simulink model "F16ASYM_Controlled"  (R2015a)
settings: Solver=ode3  SolverMode=SingleTasking  StartTime=0.0  StopTime=inf  FixedStep=T_sim  RelTol=1e-3
InitFcn:
  | load('NN_c_weights_Last_stable.mat')
StopFcn:
  | Final_results
values from neighbouring files (symbols this model uses):
  a1 = fitresult.p1    [Stall_protection.m]
  alpha_map_eval = ones(size(M_eval))*NaN    [Auto_trim_aid.m]    (also in Autotrim_maps.mat = [nan nan 0.277598136245 0.119432432992 0.0579479097061 0.027)
  beta_map_eval = ones(size(M_eval))*NaN    [Auto_trim_aid.m]    (also in Autotrim_maps.mat = [nan nan -0.00151549403324 0.00117807579006 -0.0052086799721)
  C_L_0 = fitresult.p2    [Stall_protection.m]
  G_eval = NaN*ones(size(M_sq,2),size(H_sq,2))    [Stall_protection.m]
  H_sq = unique(sort(H_sq))    [Stall_protection.m]
  H_sq_autotrim = min( F_envelope.H_1g):2000:max(F_envelope.H_1g)    [Auto_trim_aid.m]    (also in Autotrim_maps.mat = [0 2000 4000 6000 8000 10000 12000 14000 16000 18000])
  K_b_q_extrap_ACC = K_b_q_extrap    [RUN_ME.m]
  K_b_q_extrap_AoA = K_b_q_extrap    [RUN_ME.m]
  M_sq = unique(sort(M_sq))    [Stall_protection.m]
  M_sq_autotrim = 0:0.1:max(F_envelope.M_1g)    [Auto_trim_aid.m]    (also in Autotrim_maps.mat = [0 0.1 0.2 0.3 0.4 0.5 0.6 0.7 0.8 0.9 1 1.1 ... (21 element)
  T_sim = 0.02    [RUN_ME.m]
  tau_q_extrap_ACC = tau_q_extrap    [RUN_ME.m]
  tau_q_extrap_AoA = tau_q_extrap    [RUN_ME.m]
  velocity = M_eval(I,J)*a    [Auto_trim_aid.m]
undefined symbols (not defined in the file or in its folder): ACCEL, B, Earth, fi_flag_Simulink, GYRO, H_sq_sche, k_B, K_b_ACC_extrap, K_b_AoA_extrap, latitude, longitude, m, m_B, M_sq_sche, Model_used_flag, rad, s, sigbuilder_block, Stall_curve, tau_ACC_extrap, tau_AoA_extrap, Theta_1_roll_last, Theta_2_roll_last, Theta_3_roll_last, trim_control, trim_state, trim_throttle, V_Comp_A_w_z_last, V_Comp_last, V_Comp_last_ONE, V_long_lastA_w_z, V_long_lastAoA, V_roll_last, V_roll_lastMOD, V_yaw_last, W_Comp_A_w_z_last, W_Comp_last, W_long_lastA_w_z, W_long_lastAoA, W_roll_last, W_roll_lastMOD, W_yaw_last, WGS84
libraries: Adaptive_FaultTolerantControl x57, dspsigops x37, F16_Actuator_Library x14, commnoisgen2 x13, simulink x11, simulink_extras x10, dsparch4 x6, aerolibatmos2 x6, aerolibtransform2 x6, aerolibfltsims x3, dspvision x3, dspsnks4 x3
(part 4 of 14)

== system F16ASYM_Controlled/Sensors and filtering/Sensors and filtering. No noise ==
  note: This is measured load factor
  state : Inport
  Bus Creator : BusCreator  Inputs=8
  Bus Selector2 : BusSelector  OutputSignals=X_e,TAS,alpha ; beta,p;q;r,euler,an_b_CG,Throttle
  Demux : Demux  Outputs=3
  Demux1 : Demux  Outputs=2
  Gain{1..8} (8 alike) : Gain
  Terminator : Terminator
  Terminator1 : Terminator
  All_measures : Outport
  wires:
  state/1 -> Bus Selector2/1
  Bus Selector2/1 -> Demux/1  "<X_e>"
  Gain8/1 -> Bus Creator/1  "Alt meas (m)"
  Demux/1 -> Terminator/1
  Demux/2 -> Terminator1/1
  Bus Selector2/2 -> Gain7/1  "<TAS>"
  Bus Selector2/3 -> Demux1/1  "<alpha ; beta>"
  Gain5/1 -> Bus Creator/3  "AoA meas (rad)"
  Gain6/1 -> Bus Creator/4  "SS meas (rad)"
  Bus Selector2/4 -> Gain3/1  "<p;q;r>"
  Bus Selector2/5 -> Gain2/1  "<euler>"
  Bus Selector2/6 -> Gain1/1  "<an_b_CG>"
  Gain7/1 -> Bus Creator/2  "V_TAS (m/s)"
  Gain3/1 -> Bus Creator/5  "omega_b meas (rad/s)"
  Bus Creator/1 -> All_measures/1
  Bus Selector2/7 -> Gain4/1  "<Throttle>"
  Gain4/1 -> Bus Creator/8  "Throttle_meas"
  Demux/3 -> Gain8/1  "Alt meas (m)"
  Demux1/2 -> Gain6/1  "SS meas (rad)"
  Demux1/1 -> Gain5/1  "AoA meas (rad)"
  Gain2/1 -> Bus Creator/6  "Euler meas (rad)"
  Gain1/1 -> Bus Creator/7  "an_b_CG meas (m/s^2)"

== system F16ASYM_Controlled/Sensors and filtering/Sensors and filtering. Noise ==
  note: This is measured load factor
  state : Inport
  "  2" : Sum  Inputs=++|
  1st order model1 : Subsystem  mask{tau=T_sim*1.4, y_i=trim_state(10:12)}
      mask prompts: tau "1st order time constant (tau)"; y_i "Initial state"
      mask init:
      | K_ref=1/tau;
      mask Display:
      | [y,t]=step(tf([K_ref],[1 K_ref]));
      | pos = get_param(gcb, 'Position');
      | width = pos(3) - pos(1);
      | height = pos(4) - pos(2);
      | t = t.*width/max(t);
      | y=y.*height/max(y);
      | plot(t,y);
      | 
      | 
      | text(0.5*width,0.92*height,['tau=',num2str(tau)]);
      | 
      | dpoly([K_ref],[1 K_ref], 's')
  1st order model2 : Subsystem  mask{tau=T_sim*1.4, y_i=trim_state(9)}
      mask prompts: tau "1st order time constant (tau)"; y_i "Initial state"
      mask init:
      | K_ref=1/tau;
      mask Display:
      | [y,t]=step(tf([K_ref],[1 K_ref]));
      | pos = get_param(gcb, 'Position');
      | width = pos(3) - pos(1);
      | height = pos(4) - pos(2);
      | t = t.*width/max(t);
      | y=y.*height/max(y);
      | plot(t,y);
      | 
      | 
      | text(0.5*width,0.92*height,['tau=',num2str(tau)]);
      | 
      | dpoly([K_ref],[1 K_ref], 's')
  1st order model3 : Subsystem  mask{tau=T_sim*1.4, y_i=trim_state(8)}
      mask prompts: tau "1st order time constant (tau)"; y_i "Initial state"
      mask init:
      | K_ref=1/tau;
      mask Display:
      | [y,t]=step(tf([K_ref],[1 K_ref]));
      | pos = get_param(gcb, 'Position');
      | width = pos(3) - pos(1);
      | height = pos(4) - pos(2);
      | t = t.*width/max(t);
      | y=y.*height/max(y);
      | plot(t,y);
      | 
      | 
      | text(0.5*width,0.92*height,['tau=',num2str(tau)]);
      | 
      | dpoly([K_ref],[1 K_ref], 's')
  Add : Sum  Inputs=|++
  Add1 : Sum  Inputs=|++
  Add2 : Sum  Inputs=++|
  Add3 : Sum  Inputs=|++
  Bus Creator : BusCreator  Inputs=8
  Bus Selector2 : BusSelector  OutputSignals=X_e,TAS,alpha ; beta,p;q;r,an_b_CG,euler,Throttle
  Delay : Delay  DelayLength=5  InitialCondition=trim_state(4:6)
  Demux : Demux  Outputs=3
  Demux1 : Demux  Outputs=2
  Gain4 : Gain
  Gaussian Noise Generator4 : commnoisgen2/Gaussian Noise Generator  m=deg2rad(0.003)/3600  d=1.2e-9*eye(3,3)  s=41  Ts=T_sim  frameBased=off  sampPerFrame=1  orient=off  outDataType=double
  Inertial Measurement Unit : Subsystem
  Scope : Scope
      settings: YMin=-250  YMax=4250  SaveName=ScopeData40
  Scope1 : Scope
      settings: YMin=-0.3  YMax=1.8  SaveName=ScopeData41
  Terminator : Terminator
  Terminator1 : Terminator
  "Uniform Noise " : commnoisgen2/Uniform Noise Generator  low=-0.05  up=0.05  seed=31  Ts=T_sim  frameBased=off  sampPerFrame=1  orient=off  outDataType=double
  Uniform Noise Generator : commnoisgen2/Uniform Noise Generator  low=-10  up=10  seed=31  Ts=T_sim  frameBased=off  sampPerFrame=1  orient=off  outDataType=double
  Uniform Noise Generator2 : commnoisgen2/Uniform Noise Generator  low=-deg2rad(0.2)  up=deg2rad(0.2)  seed=31  Ts=T_sim  frameBased=off  sampPerFrame=1  orient=off  outDataType=double
  Uniform Noise Generator3 : commnoisgen2/Uniform Noise Generator  low=-deg2rad(0.2)  up=deg2rad(0.2)  seed=31  Ts=T_sim  frameBased=off  sampPerFrame=1  orient=off  outDataType=double
  All_measures : Outport
  wires:
  state/1 -> Bus Selector2/1
  Bus Selector2/1 -> Demux/1  "<X_e>"
  Add/1 -> Bus Creator/1  "Alt meas (m)"
  Demux/1 -> Terminator/1
  Demux/2 -> Terminator1/1
  Bus Selector2/2 -> Add1/1  "<TAS>"
  Bus Selector2/3 -> Demux1/1  "<alpha ; beta>"
  Add2/1 -> 1st order model3/1(y_in)  "AoA meas (rad)"
  1st order model2/1(y_out) -> Bus Creator/4  "SS meas (rad)"
  Bus Selector2/6 -> "  2"/2  "<euler>"
  Add1/1 -> Bus Creator/2  "V_TAS (m/s)"
  Inertial Measurement Unit/1(measured angular rate) -> 1st order model1/1(y_in)  "omega_b meas (rad/s)"
  "  2"/1 -> Delay/1
  Inertial Measurement Unit/2(measured acceleration) -> Bus Creator/6  "an_b_CG meas (m/s^2)"
  Bus Creator/1 -> Scope/1, All_measures/1
  Bus Selector2/7 -> Gain4/1  "<Throttle>"
  Gain4/1 -> Bus Creator/8  "Throttle_meas"
  Demux/3 -> Add/1  "Alt meas (m)"
  Demux1/2 -> Add3/1  "SS meas (rad)"
  Demux1/1 -> Add2/2  "AoA meas (rad)"
  Delay/1 -> Bus Creator/7  "Euler meas (rad)"
  Uniform Noise Generator/1 -> Add/2
  "Uniform Noise "/1 -> Add1/2
  Uniform Noise Generator2/1 -> Add2/1
  Uniform Noise Generator3/1 -> Add3/2
  Gaussian Noise Generator4/1 -> "  2"/1
  Bus Selector2/4 -> Inertial Measurement Unit/1(real angular rate)  "<p;q;r>"
  Bus Selector2/5 -> Inertial Measurement Unit/2(real acceleration)  "<an_b_CG>"
  1st order model1/1(y_out) -> Bus Creator/5, Scope1/1  "omega_b meas (rad/s)"
  1st order model3/1(y_out) -> Bus Creator/3  "AoA meas (rad)"
  Add3/1 -> 1st order model2/1(y_in)

== system F16ASYM_Controlled/Speed-Throttle control/Stall protection TAS ==
  TAS comm : Inport
  All meas : Inport  Port=2
  Add : Sum  Inputs=+-
  Bus Selector : BusSelector  OutputSignals=signal1.V_TAS (m/s),signal1.Alt meas (m),signal2.a
  Compare To Zero : simulink/Logic and Bit Operations/Compare To Zero  relop=>=  OutDataTypeStr=boolean
  Display : Display
  Min TAS : Product  Inputs=**
  MinMax : MinMax  Function=max  Inputs=2
  Stall curve 1g : Lookup_n-D  NumberOfTableDimensions=1  BreakpointsForDimension1=Stall_curve.H_2  Table=Stall_curve.M_2  RemoveProtectionInput=on  RndMeth=Simplest  InputSameDT=on
  Stop Simulation : Stop
  margin : Gain  Gain=1.2
  TAS des : Outport
  tag scope: Min_Mach=global
  wires:
  MinMax/1 -> TAS des/1
  TAS comm/1 -> MinMax/2
  All meas/1 -> Bus Selector/1
  Bus Selector/2 -> Stall curve 1g/1  "<Alt meas (m)>"
  Stall curve 1g/1 -> [Min_Mach], Min TAS/1  "Min M"
  Bus Selector/3 -> Min TAS/2  "<a>"
  Min TAS/1 -> Add/1, margin/1
  margin/1 -> MinMax/1
  Add/1 -> Display/1, Compare To Zero/1
  Compare To Zero/1 -> Stop Simulation/1
  Bus Selector/1 -> Add/2  "<V_TAS (m/s)>"

== system F16ASYM_Controlled/Speed-Throttle control/Throttle controller ==
  V_TAS des : Inport
  All meas : Inport  Port=2
  Add : Sum  Inputs=|+-
  Bus Selector : BusSelector  OutputSignals=signal1.V_TAS (m/s)
  Mux : Mux  Inputs=2
  PID Controller2 : simulink/Continuous/PID Controller  Controller=P  TimeDomain=Continuous-time  SampleTime=-1  IntegratorMethod=Forward Euler  FilterMethod=Forward Euler  Form=Parallel  UseFilter=on  ControllerParametersSource=internal  P=0.8  I=0.0001  D=-0.01  N=100  InitialConditionSource=internal  InitialConditionForIntegrator=0  InitialConditionForFilter=0  ExternalReset=none  LimitOutput=on  UpperSaturationLimit=1  LowerSaturationLimit=0  LinearizeAsGain=on  AntiWindupMode=back-calculation  Kb=3  TrackingMode=off  Kt=1  PParamMin=[]  PParamMax=[]  IParamMin=[]  IParamMax=[]  DParamMin=[]  DParamMax=[]  NParamMin=[]  NParamMax=[]  KbParamMin=[]  KbParamMax=[]  KtParamMin=[]  KtParamMax=[]  POutMin=[]  POutMax=[]  IOutMin=[]  IOutMax=[]  DOutMin=[]  DOutMax=[]  NOutMin=[]  NOutMax=[]  KbOutMin=[]  KbOutMax=[]  KtOutMin=[]  KtOutMax=[]  IntegratorOutMin=[]  IntegratorOutMax=[]  FilterOutMin=[]  FilterOutMax=[]  SumOutMin=[]  SumOutMax=[]  SumI1OutMin=[]  SumI1OutMax=[]  SumI2OutMin=[]  SumI2OutMax=[]  SumI3OutMin=[]  SumI3OutMax=[]  SumDOutMin=[]  SumDOutMax=[]  SaturationOutMin=[]  SaturationOutMax=[]  IntegratorContinuousStateAttributes=''  IntegratorStateMustResolveToSignalObject=off  IntegratorRTWStateStorageClass=Auto  FilterContinuousStateAttributes=''  FilterStateMustResolveToSignalObject=off  FilterRTWStateStorageClass=Auto  DifferentiatorICPrevScaledInput=0  DifferentiatorOutMin=[]  DifferentiatorOutMax=[]
  Scope : Scope
      settings: YMin=152.5  YMax=207.5  SaveName=ScopeData30
  Scope1 : Scope
      settings: YMin=1  YMax=1  SaveName=ScopeData31
  Throttle des : Outport
  wires:
  All meas/1 -> Bus Selector/1
  V_TAS des/1 -> Mux/1, Add/1
  Bus Selector/1 -> Mux/2, Add/2  "<V_TAS (m/s)>"
  PID Controller2/1 -> Scope1/1, Throttle des/1
  Add/1 -> PID Controller2/1
  Mux/1 -> Scope/1

== system F16ASYM_Controlled/Stall protection A_z and AoA/AoA and load factor map ==
  Control in : Inport
  Reconf param : Inport  Port=2
  All meas : Inport  Port=3
  A_w_z comm : Inport  Port=4
  AoA comm : Inport  Port=5
  2-D Lookup Table : Lookup_n-D  BreakpointsForDimension1=M_sq  BreakpointsForDimension2=H_sq  Table=G_eval  RemoveProtectionInput=on  SampleTime=5*T_sim  RndMeth=Simplest  InputSameDT=on
  Bias : Bias  Bias=1
  Bus Selector : BusSelector  OutputSignals=signal2.Mach,signal1.Alt meas (m),signal1.AoA meas (rad),signal2.A_w_CG
  Constant : Constant  Value=0
  Display : Display
  Display1 : Display
  Gain : Gain  Gain=-1
  Gain1 : Gain  Gain=-1
  Gain2 : Gain  Gain=9.81
  If : If  NumInputs=4  IfExpression=u1>=17 | (u1<=-17) | (u2>=u3) | (u2<=u4)  SampleTime=T_sim
  If Action Subsystem : Subsystem  TreatAsAtomicUnit=on
  Radians to Degrees : simulink_extras/Transformations/Radians to Degrees
  Rate Limiter : RateLimiter  RisingSlewLimit=2*9.8  FallingSlewLimit=-2*9.8  SampleTimeMode=inherited
  Rate Limiter2 : RateLimiter  RisingSlewLimit=deg2rad(15)  FallingSlewLimit=-deg2rad(15)  SampleTimeMode=inherited  InitialCondition=trim_state(8)
  Saturation : Saturate  UpperLimit=deg2rad(20)  LowerLimit=-deg2rad(20)
  Saturation Dynamic : simulink/Discontinuities/Saturation Dynamic  OutMin=[]  OutMax=[]  OutDataTypeStr=Inherit: Same as second input  OutDataType=fixdt(1, 16)  OutScaling=2^-10  DoSatur=off
  Saturation1 : Saturate  UpperLimit=10  LowerLimit=0
  Selector : Selector  InputPortWidth=3  Indices=3
  Switch : Switch  Threshold=0.5
  Terminator : Terminator
  Terminator1 : Terminator
  isNaN1 : RelationalOperator  Operator=isNaN  OutDataTypeStr=boolean
  A_w_z des : Outport
  AoA des : Outport  Port=2
  wires:
  If/1 -> If Action Subsystem/Action
  Switch/1 -> Gain/1, Saturation Dynamic/1, If/3, Display/1
  Constant/1 -> Switch/1
  isNaN1/1 -> Switch/2
  Gain2/1 -> isNaN1/1, Switch/3
  Saturation1/1 -> Gain2/1
  Gain1/1 -> Display1/1, If/2
  Selector/1 -> Gain1/1
  Bus Selector/4 -> Selector/1  "<A_w_CG>"
  Radians to Degrees/1 -> If/1
  Bus Selector/3 -> Radians to Degrees/1  "<AoA meas (rad)>"
  Gain/1 -> Saturation Dynamic/3, If/4
  Bias/1 -> Saturation1/1
  Saturation Dynamic/1 -> A_w_z des/1
  Rate Limiter/1 -> Saturation Dynamic/2
  Rate Limiter2/1 -> AoA des/1
  AoA comm/1 -> Saturation/1
  Bus Selector/1 -> 2-D Lookup Table/1  "<Mach>"
  2-D Lookup Table/1 -> Bias/1
  Bus Selector/2 -> 2-D Lookup Table/2  "<Alt meas (m)>"
  A_w_z comm/1 -> Rate Limiter/1
  Saturation/1 -> Rate Limiter2/1
  All meas/1 -> Bus Selector/1
  Control in/1 -> Terminator/1
  Reconf param/1 -> Terminator1/1

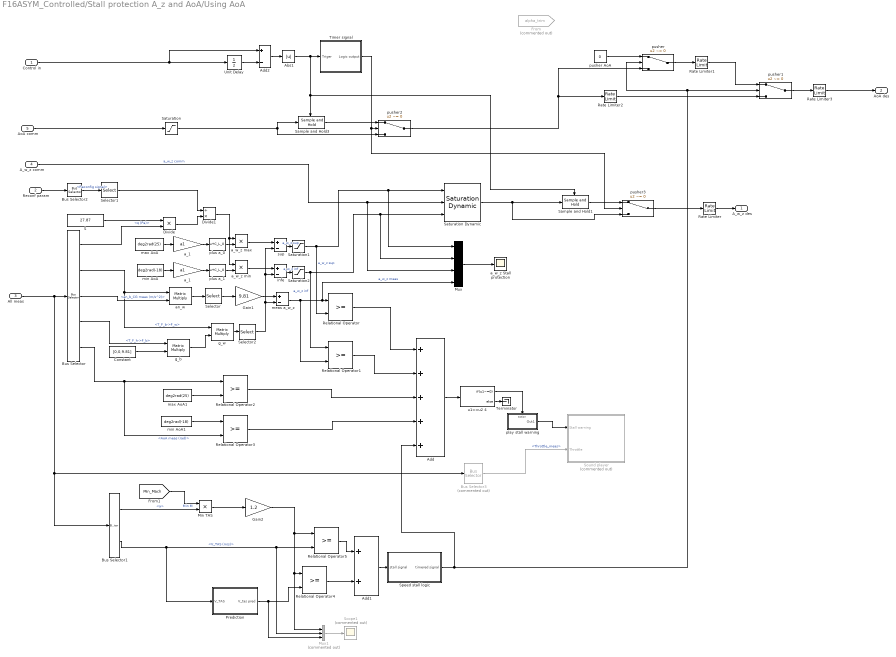
== system F16ASYM_Controlled/Stall protection A_z and AoA/Using AoA ==
  Control in : Inport
  Reconf param : Inport  Port=2
  All meas : Inport  Port=3
  A_w_z comm : Inport  Port=4
  AoA comm : Inport  Port=5
  Abs1 : Abs
  Add : Sum  Inputs=+++++
  Add1 : Sum
  Add2 : Sum  Inputs=+-  OutDataTypeStr=double
  Bus Selector : BusSelector  OutputSignals=signal2.q (Pa),signal2.T_F_b->F_w,signal1.an_b_CG meas (m/s^2),signal2.T_F_h->F_b,signal1.AoA meas (rad)
  Bus Selector1 : BusSelector  OutputSignals=signal2.a,signal1.V_TAS (m/s)
  Bus Selector2 : BusSelector  OutputSignals=Reconfig signal
  Bus Selector3 : BusSelector  Commented=on  OutputSignals=signal1.Throttle_meas
  Constant : Constant  Value=[0,0,9.81]
  Divide : Product  Inputs=**
  Divide1 : Product  Inputs=/*
  From : From  Commented=on  GotoTag=alpha_trim  TagVisibility=global
  Gain1 : Gain  Gain=9.81
  Gain2 : Gain  Gain=1.2
  Min TAS : Product  Inputs=**
  Mux : Mux
  Mux1 : Mux  Commented=on  Inputs=3
  Prediction : Subsystem  mask{T_pred=2}
      mask prompts: T_pred "Prediction time"
      mask TypeOptions T_pred: T_pred/Gain
  Rate Limiter : RateLimiter  RisingSlewLimit=6*9.8  FallingSlewLimit=-6*9.8  SampleTimeMode=inherited
  Rate Limiter1 : RateLimiter  RisingSlewLimit=deg2rad(2)  FallingSlewLimit=-deg2rad(2)  SampleTimeMode=inherited  InitialCondition=trim_state(8)
  Rate Limiter2 : RateLimiter  RisingSlewLimit=deg2rad(10)  FallingSlewLimit=-deg2rad(10)  SampleTimeMode=inherited  InitialCondition=trim_state(8)
  Rate Limiter3 : RateLimiter  RisingSlewLimit=deg2rad(10)  FallingSlewLimit=-deg2rad(10)  SampleTimeMode=inherited  InitialCondition=trim_state(8)
  Relational Operator{,1..5} (6 alike) : RelationalOperator  OutDataTypeStr=boolean
  S : Constant  Value=27.87
  Sample and Hold1 : dspsigops/Sample and Hold  trig=Either edge  initCond=0  latchinput=off
  Sample and Hold3 : dspsigops/Sample and Hold  trig=Either edge  initCond=0  latchinput=off
  Saturation : Saturate  UpperLimit=deg2rad(25)  LowerLimit=-deg2rad(19)
  Saturation Dynamic : simulink/Discontinuities/Saturation Dynamic  OutMin=[]  OutMax=[]  OutDataTypeStr=Inherit: Same as second input  OutDataType=fixdt(1, 16)  OutScaling=2^-10  DoSatur=off
  Saturation1 : Saturate  UpperLimit=9*9.81  LowerLimit=0
  Saturation2 : Saturate  UpperLimit=0  LowerLimit=-4*9.81
  Scope1 : Scope  Commented=on
      settings: YMin=80  YMax=210  SaveName=ScopeData25
  Selector : Selector  InputPortWidth=3  Indices=3
  Selector1 : Selector  InputPortWidth=19
  Selector2 : Selector  InputPortWidth=3  Indices=3
  Sound player : Subsystem  Commented=on
  Speed stall logic : Subsystem
  Terminator : Terminator
  Timer signal : Subsystem  mask{time_delay=1.5}
      mask prompts: time_delay "Time to delay (s)"
  Unit Delay : UnitDelay  SampleTime=-1
  a_1 : Gain  Gain=a1
  "a_1  " : Gain  Gain=a1
  a_w_z Stall protection : Scope
      settings: ShowLegends=on  TimeRange=8.515176374077115  YMin=25.2511160714286  YMax=100  SaveName=ScopeData28
  a_w_z max : Product  Inputs=**
  a_w_z min : Product  Inputs=**
  an_w : Product  Multiplication=Matrix(*)
  g_b : Product  Multiplication=Matrix(*)
  g_w : Product  Multiplication=Matrix(*)
  infe : Sum  Inputs=+-
  max AoA : Constant  Value=deg2rad(25)
  max AoA1 : Constant  Value=deg2rad(25)
  meas a_w_z : Sum  Inputs=+-
  min AoA : Constant  Value=deg2rad(-18)
  min AoA1 : Constant  Value=deg2rad(-18)
  play stall warning : Subsystem  TreatAsAtomicUnit=on
  plus a_0 : Bias  Bias=C_L_0
  plus a_1 : Bias  Bias=C_L_0
  pusher{,1..3} (4 alike) : Switch  Criteria=u2 ~= 0  Threshold=0.5
  pusher AoA : Constant  Value=0
  sup : Sum  Inputs=+-
  u1>=u2 4 : If  IfExpression=u1~=0  SampleTime=T_sim*2
  A_w_z des : Outport
  AoA des : Outport  Port=2
  wires:
  AoA comm/1 -> Saturation/1
  pusher1/1 -> Rate Limiter3/1
  A_w_z comm/1 -> Mux/3, Saturation Dynamic/2  "a_w_z comm"
  All meas/1 -> Bus Selector1/1, Bus Selector3/1, Bus Selector/1
  [Min_Mach] -> Min TAS/1  "Min M"
  Bus Selector1/1 -> Min TAS/2  "<a>"
  Reconf param/1 -> Bus Selector2/1
  S/1 -> Divide/1
  Bus Selector/1 -> Divide/2  "<q (Pa)>"
  Bus Selector2/1 -> Selector1/1  "<Reconfig signal>"
  Selector1/1 -> Divide1/1
  Divide/1 -> Divide1/2
  a_1/1 -> plus a_0/1
  Divide1/1 -> a_w_z min/1, a_w_z max/1
  plus a_0/1 -> a_w_z max/2
  Bus Selector/3 -> an_w/2  "<an_b_CG meas (m/s^2)>"
  Bus Selector/2 -> g_w/1, an_w/1  "<T_F_b->F_w>"
  Selector/1 -> Gain1/1
  an_w/1 -> Selector/1
  Bus Selector/4 -> g_b/1  "<T_F_h->F_b>"
  Constant/1 -> g_b/2
  g_b/1 -> g_w/2
  a_w_z max/1 -> sup/1
  g_w/1 -> Selector2/1
  Gain1/1 -> meas a_w_z/1
  Rate Limiter/1 -> A_w_z des/1
  a_w_z min/1 -> infe/1
  Selector2/1 -> meas a_w_z/2, infe/2, sup/2
  "a_1  "/1 -> plus a_1/1
  plus a_1/1 -> a_w_z min/2
  max AoA/1 -> a_1/1
  min AoA/1 -> "a_1  "/1
  sup/1 -> Saturation1/1  "a_w_z sup"
  infe/1 -> Saturation2/1  "a_w_z inf"
  Bus Selector/5 -> Relational Operator3/2, Relational Operator2/1  "<AoA meas (rad)>"
  max AoA1/1 -> Relational Operator2/2
  min AoA1/1 -> Relational Operator3/1
  Mux/1 -> a_w_z Stall protection/1
  Bus Selector1/2 -> Mux1/2, Relational Operator5/2, Prediction/1(V_TAS)  "<V_TAS (m/s)>"
  Gain2/1 -> Mux1/1, Relational Operator4/1, Relational Operator5/1
  Relational Operator/1 -> Add/1
  Relational Operator1/1 -> Add/2
  Relational Operator2/1 -> Add/3
  Relational Operator3/1 -> Add/4
  u1>=u2 4/1 -> play stall warning/Action
  meas a_w_z/1 -> Relational Operator1/2, Mux/4, Relational Operator/1  "a_w_z meas"
  Add/1 -> u1>=u2 4/1
  pusher2/1 -> pusher/3, Rate Limiter2/1
  Saturation1/1 -> Relational Operator/2, Mux/1, Saturation Dynamic/1  "a_w_z sup"
  Saturation2/1 -> Relational Operator1/1, Mux/2, Saturation Dynamic/3  "a_w_z inf"
  Min TAS/1 -> Gain2/1
  Prediction/1(V_tas pred) -> Mux1/3, Relational Operator4/2
  Add1/1 -> Speed stall logic/1(stall signal)
  Mux1/1 -> Scope1/1
  Speed stall logic/1(timered signal) -> pusher/2, pusher1/2, Add/5
  pusher/1 -> Rate Limiter1/1
  Rate Limiter2/1 -> pusher1/3
  Rate Limiter1/1 -> pusher1/1
  Unit Delay/1 -> Add2/2
  Control in/1 -> Add2/1, Unit Delay/1
  Abs1/1 -> Sample and Hold3/Trigger, Sample and Hold1/Trigger, Timer signal/1(Triger)
  Add2/1 -> Abs1/1
  Saturation/1 -> Sample and Hold3/1, pusher2/3
  Sample and Hold3/1 -> pusher2/1
  Saturation Dynamic/1 -> pusher3/3, Sample and Hold1/1
  Timer signal/1(Logic output) -> pusher2/2, pusher3/2
  Sample and Hold1/1 -> pusher3/1
  pusher3/1 -> Rate Limiter/1
  pusher AoA/1 -> pusher/1
  Rate Limiter3/1 -> AoA des/1
  u1>=u2 4/2 -> Terminator/1
  play stall warning/1(Out1) -> Sound player/1(Stall warning)
  Bus Selector3/1 -> Sound player/2(Throttle)  "<Throttle_meas>"
  Relational Operator4/1 -> Add1/2
  Relational Operator5/1 -> Add1/1

== system F16ASYM_Controlled/Anti-windup Calculation/Anti-windup: NO reconfigurable/Moments ==
  C_L : Inport
  C_M : Inport  Port=2
  C_N : Inport  Port=3
  q : Inport  Port=4
  B span : Constant  Value=9.144
  CMA : Constant  Value=3.45
  Divide : Product  Inputs=**
  Divide1 : Product  Inputs=***
  Divide2 : Product  Inputs=**
  Divide3 : Product  Inputs=***
  Divide4 : Product  Inputs=**
  S_w : Constant  Value=27.87
  S_w1 : Constant  Value=27.87
  q1 : InportShadow  Port=4
  L : Outport
  M : Outport  Port=2
  N : Outport  Port=3
  wires:
  Divide4/1 -> M/1  "M"
  Divide3/1 -> Divide4/2
  C_M/1 -> Divide4/1
  CMA/1 -> Divide3/3
  S_w1/1 -> Divide3/2
  q1/1 -> Divide3/1
  Divide2/1 -> N/1  "N"
  C_N/1 -> Divide2/2
  Divide/1 -> L/1  "L"
  Divide1/1 -> Divide/2, Divide2/1
  C_L/1 -> Divide/1
  B span/1 -> Divide1/3
  S_w/1 -> Divide1/2
  q/1 -> Divide1/1

== system F16ASYM_Controlled/Anti-windup Calculation/Anti-windup: Reconfigurable/Moments ==
  C_L : Inport
  C_M : Inport  Port=2
  C_N : Inport  Port=3
  q : Inport  Port=4
  B span : Constant  Value=9.144
  CMA : Constant  Value=3.45
  Divide : Product  Inputs=**
  Divide1 : Product  Inputs=***
  Divide2 : Product  Inputs=**
  Divide3 : Product  Inputs=***
  Divide4 : Product  Inputs=**
  S_w : Constant  Value=27.87
  S_w1 : Constant  Value=27.87
  q1 : InportShadow  Port=4
  L : Outport
  M : Outport  Port=2
  N : Outport  Port=3
  wires:
  Divide4/1 -> M/1  "M"
  Divide3/1 -> Divide4/2
  C_M/1 -> Divide4/1
  CMA/1 -> Divide3/3
  S_w1/1 -> Divide3/2
  q1/1 -> Divide3/1
  Divide2/1 -> N/1  "N"
  C_N/1 -> Divide2/2
  Divide/1 -> L/1  "L"
  Divide1/1 -> Divide/2, Divide2/1
  C_L/1 -> Divide/1
  B span/1 -> Divide1/3
  S_w/1 -> Divide1/2
  q/1 -> Divide1/1

== system F16ASYM_Controlled/Control allocator/Control allocator: NO RECONF/Leading Edge Flap:Symetric deflection ==
  note: Initialize LF_state with -alpha0 value in degrees!!!!
  note: Same as atmos() in nlplant...c
  note: see NASA Technical Paper 1538, p34
  All_meas : Inport
  Bus Selector : BusSelector  OutputSignals=signal1.Alt meas (m),signal1.V_TAS (m/s),signal1.AoA meas (rad)
  Creating    qbar / ps : Subsystem
  Gain : Gain  Gain=2  SaturateOnIntegerOverflow=on  OutDataTypeStr=Inherit: Same as input  ParamDataTypeStr=Inherit: Same as input
  Gain1 : Gain  Gain=7.25  SaturateOnIntegerOverflow=on  OutDataTypeStr=Inherit: Same as input  ParamDataTypeStr=Inherit: Same as input
  Gain2 : Gain  Gain=1.38  SaturateOnIntegerOverflow=on  OutDataTypeStr=Inherit: Same as input  ParamDataTypeStr=Inherit: Same as input
  LF_state : Integrator  InitialCondition=-trim_state(8)*180/pi
  Sum : Sum  Inputs=-|+|+  SaturateOnIntegerOverflow=on  InputSameDT=on  OutDataTypeStr=Inherit: Same as first input
  Sum1 : Sum  Inputs=|+-  SaturateOnIntegerOverflow=on  InputSameDT=on  OutDataTypeStr=Inherit: Same as first input
  Sum2 : Sum  Inputs=++|  SaturateOnIntegerOverflow=on  InputSameDT=on  OutDataTypeStr=Inherit: Same as first input
  coeff1 : Constant  Value=1.45
  r2d1 : Gain  Gain=180/pi  SaturateOnIntegerOverflow=on  OutDataTypeStr=Inherit: Same as input  ParamDataTypeStr=Inherit: Same as input
  r2d6 : Gain  Gain=9.05  SaturateOnIntegerOverflow=on  OutDataTypeStr=Inherit: Same as input  ParamDataTypeStr=Inherit: Same as input
  delta_lef (deg) : Outport
  wires:
  Bus Selector/3 -> r2d1/1  "<AoA meas (rad)>"
  Bus Selector/1 -> Creating    qbar / ps/1(alt)  "<Alt meas (m)>"
  r2d6/1 -> Sum/1
  Creating    qbar / ps/1(qbar / ps) -> r2d6/1
  Bus Selector/2 -> Creating    qbar / ps/2(V)  "<V_TAS (m/s)>"
  r2d1/1 -> Gain/1, Sum1/1  "alpha deg"
  LF_state/1 -> Sum2/2
  Sum2/1 -> Gain2/1, Sum1/2
  coeff1/1 -> Sum/3
  Gain2/1 -> Sum/2
  Gain/1 -> Sum2/1
  Gain1/1 -> LF_state/1
  Sum1/1 -> Gain1/1
  All_meas/1 -> Bus Selector/1
  Sum/1 -> delta_lef (deg)/1

== system F16ASYM_Controlled/Control allocator/Control allocator: RECONFIG/Blockades logic: Limits injetor ==
  note: 1st order models here to avoid coupling
  note: No dynamics for throttle since the engine dynamics is inside the model
  Abs pos limits : Inport
  Last deflection (abs) : Inport  Port=2
  Blockades : Inport  Port=3
  Blockade now : Inport  Port=4
  1st order model : Subsystem  mask{tau=T_sim*4, y_i=[-24,-24,-21,-21,-29,0,0]}
      mask prompts: tau "1st order time constant (tau)"; y_i "Initial state"
      mask init:
      | K_ref=1/tau;
      mask Display:
      | [y,t]=step(tf([K_ref],[1 K_ref]));
      | pos = get_param(gcb, 'Position');
      | width = pos(3) - pos(1);
      | height = pos(4) - pos(2);
      | t = t.*width/max(t);
      | y=y.*height/max(y);
      | plot(t,y);
      | 
      | 
      | text(0.5*width,0.92*height,['tau=',num2str(tau)]);
      | 
      | dpoly([K_ref],[1 K_ref], 's')
  1st order model1 : Subsystem  mask{tau=T_sim*4, y_i=[24,24,21,21,29,25,25]}
      mask prompts: tau "1st order time constant (tau)"; y_i "Initial state"
      mask init:
      | K_ref=1/tau;
      mask Display:
      | [y,t]=step(tf([K_ref],[1 K_ref]));
      | pos = get_param(gcb, 'Position');
      | width = pos(3) - pos(1);
      | height = pos(4) - pos(2);
      | t = t.*width/max(t);
      | y=y.*height/max(y);
      | plot(t,y);
      | 
      | 
      | text(0.5*width,0.92*height,['tau=',num2str(tau)]);
      | 
      | dpoly([K_ref],[1 K_ref], 's')
  Add : Sum
  Block AT INFERIOR LIMIT : Subsystem
  Block AT SUPERIOR LIMIT : Subsystem
  Block NOW INFERIOR LIMIT : Subsystem
  Block NOW SUPERIOR LIMIT : Subsystem
  Inf : Selector  NumberOfDimensions=2  InputPortWidth=3  IndexOptions=Index vector (dialog),Index vector (dialog)  Indices=[1:7],1  OutputSizes=1,1
  Matrix Concatenate : Concatenate  Mode=Multidimensional array  ConcatenateDimension=2
  Saturation : Saturate  UpperLimit=1  LowerLimit=0
  Sup : Selector  NumberOfDimensions=2  InputPortWidth=3  IndexOptions=Index vector (dialog),Index vector (dialog)  Indices=[1:7],2  OutputSizes=1,1
  Pos limits(abs) : Outport
  Surf blocked : Outport  Port=2
  wires:
  Last deflection (abs)/1 -> Block NOW SUPERIOR LIMIT/3(Last deflection (abs)), Block NOW INFERIOR LIMIT/3(Last deflection (abs))
  Matrix Concatenate/1 -> Pos limits(abs)/1
  Blockade now/1 -> Block NOW SUPERIOR LIMIT/2(Blockade now), Block NOW INFERIOR LIMIT/2(Blockade now), Add/2
  Abs pos limits/1 -> Sup/1, Inf/1
  Blockades/1 -> Block AT INFERIOR LIMIT/2(Blockades), Block AT SUPERIOR LIMIT/2(Blockades)
  Inf/1 -> Block AT INFERIOR LIMIT/1(Limit)
  Sup/1 -> Block AT SUPERIOR LIMIT/1(Limit)
  Block AT INFERIOR LIMIT/1(Reconfig limits) -> Block NOW INFERIOR LIMIT/1(Limit)
  Block AT SUPERIOR LIMIT/1(Reconfig limits) -> Block NOW SUPERIOR LIMIT/1(Limit)
  1st order model/1(y_out) -> Matrix Concatenate/1
  Block NOW SUPERIOR LIMIT/1(Reconfig limits) -> 1st order model1/1(y_in)
  Block AT INFERIOR LIMIT/2(Surf blocked) -> Add/1
  Add/1 -> Saturation/1
  Saturation/1 -> Surf blocked/1
  Block NOW INFERIOR LIMIT/1(Reconfig limits) -> 1st order model/1(y_in)
  1st order model1/1(y_out) -> Matrix Concatenate/2

== system F16ASYM_Controlled/Control allocator/Control allocator: RECONFIG/Leading Edge Flap:Symetric deflection ==
  note: see NASA Technical Paper 1538, p34
  note: Same as atmos() in nlplant...c
  note: Initialize LF_state with -alpha0 value in degrees!!!!
  All_meas : Inport
  Bus Selector : BusSelector  OutputSignals=signal1.Alt meas (m),signal1.V_TAS (m/s),signal1.AoA meas (rad)
  Creating    qbar / ps : Subsystem
  Gain : Gain  Gain=2  SaturateOnIntegerOverflow=on  OutDataTypeStr=Inherit: Same as input  ParamDataTypeStr=Inherit: Same as input
  Gain1 : Gain  Gain=7.25  SaturateOnIntegerOverflow=on  OutDataTypeStr=Inherit: Same as input  ParamDataTypeStr=Inherit: Same as input
  Gain2 : Gain  Gain=1.38  SaturateOnIntegerOverflow=on  OutDataTypeStr=Inherit: Same as input  ParamDataTypeStr=Inherit: Same as input
  LF_state : Integrator  InitialCondition=-trim_state(8)*180/pi
  Sum : Sum  Inputs=-|+|+  SaturateOnIntegerOverflow=on  InputSameDT=on  OutDataTypeStr=Inherit: Same as first input
  Sum1 : Sum  Inputs=|+-  SaturateOnIntegerOverflow=on  InputSameDT=on  OutDataTypeStr=Inherit: Same as first input
  Sum2 : Sum  Inputs=++|  SaturateOnIntegerOverflow=on  InputSameDT=on  OutDataTypeStr=Inherit: Same as first input
  coeff1 : Constant  Value=1.45
  r2d1 : Gain  Gain=180/pi  SaturateOnIntegerOverflow=on  OutDataTypeStr=Inherit: Same as input  ParamDataTypeStr=Inherit: Same as input
  r2d6 : Gain  Gain=9.05  SaturateOnIntegerOverflow=on  OutDataTypeStr=Inherit: Same as input  ParamDataTypeStr=Inherit: Same as input
  delta_lef (deg) : Outport
  wires:
  Sum/1 -> delta_lef (deg)/1
  All_meas/1 -> Bus Selector/1
  Sum1/1 -> Gain1/1
  Gain1/1 -> LF_state/1
  Gain/1 -> Sum2/1
  Gain2/1 -> Sum/2
  coeff1/1 -> Sum/3
  Sum2/1 -> Sum1/2, Gain2/1
  LF_state/1 -> Sum2/2
  r2d1/1 -> Sum1/1, Gain/1  "alpha deg"
  Bus Selector/2 -> Creating    qbar / ps/2(V)  "<V_TAS (m/s)>"
  Creating    qbar / ps/1(qbar / ps) -> r2d6/1
  r2d6/1 -> Sum/1
  Bus Selector/1 -> Creating    qbar / ps/1(alt)  "<Alt meas (m)>"
  Bus Selector/3 -> r2d1/1  "<AoA meas (rad)>"

== system F16ASYM_Controlled/F-16 Non-linear Plant/SYM and ASYM model: No reconfigurable/Actuators Dynamcis ==
  note: Controls:
      | 1. Throttle
      | 2. Elevator_L in deg
      | 3. Elevator_R in deg
      | 4. Aileron_L
      | 5. Aileron_R
      | 6. Rudder
      | 7. LEF_L
      | 8. LEF_R
  note: Units: deg.
  note: Units: deg.
  note: Units: deg.
  note: This addition in LEFs can be done
      |  if assumed Linear aerodynamics
  note: No dynamics for throttle since the engine dynamics is inside the model
  Control_commands : Inport
  Aileron Actuator : F16_Actuator_Library/Aileron Actuator
  Aileron Actuator1 : F16_Actuator_Library/Aileron Actuator
  Aileron_L Trim Setting : Constant  Value=trim_control(2)
  Aileron_R Trim Setting : Constant  Value=-trim_control(2)
  Control Surface Deflections : ToWorkspace  VariableName=surfaces  SampleTime=-1
      settings: Decimation=100
  Demux : Demux  Outputs=8
  Elevator Actuator : F16_Actuator_Library/Elevator Actuator
  Elevator Actuator1 : F16_Actuator_Library/Elevator Actuator
  LEF Actuator : F16_Actuator_Library/LEF Actuator
  LEF Actuator1 : F16_Actuator_Library/LEF Actuator
  Mux{,1,3..7} (7 alike) : Mux  Inputs=2
  Mux2 : Mux  Inputs=8
  Mux8 : Mux  Inputs=7
  Rudder Actuator : F16_Actuator_Library/Rudder Actuator
  Saturation1 : Saturate  UpperLimit=1  LowerLimit=0
  Control Defl Plot : Outport
  Dec_Control_def : Outport  Port=2
  Throttle_meas : Outport  Port=3
  wires:
  Saturation1/1 -> Mux2/1, Throttle_meas/1  "Throttle"
  Aileron_R Trim Setting/1 -> Aileron Actuator1/2
  Aileron_L Trim Setting/1 -> Aileron Actuator/2
  Demux/1 -> Saturation1/1
  Mux7/1 -> [LEF_R]
  LEF Actuator1/1 -> Mux7/2, Mux2/8  "LEF_R"
  Demux/8 -> Mux7/1, LEF Actuator1/1
  Mux6/1 -> [LEF_L]
  LEF Actuator/1 -> Mux2/7, Mux6/2  "LEF_L"
  Demux/7 -> Mux6/1, LEF Actuator/1
  Mux5/1 -> [Ail_R]
  Aileron Actuator1/1 -> Mux2/5, Mux5/1  "Aileron_R"
  Demux/5 -> Aileron Actuator1/1, Mux5/2
  Elevator Actuator1/1 -> Mux2/3, Mux4/1  "Elevator_R"
  Demux/3 -> Mux4/2, Elevator Actuator1/1
  Mux3/1 -> [Rudder]
  Mux1/1 -> [Ail_L]
  Rudder Actuator/1 -> Mux2/6, Mux3/2  "Rudder"
  Aileron Actuator/1 -> Mux2/4, Mux1/2  "Aileron_L"
  Demux/6 -> Mux3/1, Rudder Actuator/1
  Demux/4 -> Aileron Actuator/1, Mux1/1
  Mux/1 -> [Elev_L]
  Elevator Actuator/1 -> Mux2/2, Mux/2  "Elevator_L"
  Mux2/1 -> Control Surface Deflections/1, Dec_Control_def/1
  Demux/2 -> Elevator Actuator/1, Mux/1
  Control_commands/1 -> Demux/1
  Mux8/1 -> Control Defl Plot/1
  [Elev_L] -> Mux8/1
  [Elev_R] -> Mux8/2
  [Ail_L] -> Mux8/3
  [Ail_R] -> Mux8/4
  [Rudder] -> Mux8/5
  [LEF_L] -> Mux8/6
  [LEF_R] -> Mux8/7
  Mux4/1 -> [Elev_R]

== system F16ASYM_Controlled/F-16 Non-linear Plant/SYM and ASYM model: No reconfigurable/Leading Edge Flap:Symetric deflection ==
  note: Initialize LF_state with -alpha0 value in degrees!!!!
  note: Same as atmos() in nlplant...c
  note: see NASA Technical Paper 1538, p34
  state : Inport
  Bus Selector1 : BusSelector  OutputSignals=X_e,TAS,alpha;beta
  Creating    qbar / ps : Subsystem
  Demux1 : Demux  Outputs=2
  Gain : Gain  Gain=2  SaturateOnIntegerOverflow=on  OutDataTypeStr=Inherit: Same as input  ParamDataTypeStr=Inherit: Same as input
  Gain1 : Gain  Gain=7.25  SaturateOnIntegerOverflow=on  OutDataTypeStr=Inherit: Same as input  ParamDataTypeStr=Inherit: Same as input
  Gain2 : Gain  Gain=1.38  SaturateOnIntegerOverflow=on  OutDataTypeStr=Inherit: Same as input  ParamDataTypeStr=Inherit: Same as input
  LF_state : Integrator  InitialCondition=-trim_state(8)*180/pi
  Selector : Selector  InputPortWidth=3  Indices=3
  Sum : Sum  Inputs=-|+|+  SaturateOnIntegerOverflow=on  InputSameDT=on  OutDataTypeStr=Inherit: Same as first input
  Sum1 : Sum  Inputs=|+-  SaturateOnIntegerOverflow=on  InputSameDT=on  OutDataTypeStr=Inherit: Same as first input
  Sum2 : Sum  Inputs=++|  SaturateOnIntegerOverflow=on  InputSameDT=on  OutDataTypeStr=Inherit: Same as first input
  coeff1 : Constant  Value=1.45
  r2d1 : Gain  Gain=180/pi  SaturateOnIntegerOverflow=on  OutDataTypeStr=Inherit: Same as input  ParamDataTypeStr=Inherit: Same as input
  r2d6 : Gain  Gain=9.05  SaturateOnIntegerOverflow=on  OutDataTypeStr=Inherit: Same as input  ParamDataTypeStr=Inherit: Same as input
  delta_lef (deg) : Outport
  wires:
  Bus Selector1/3 -> Demux1/1  "<alpha;beta>"
  Bus Selector1/1 -> Selector/1  "<X_e>"
  r2d6/1 -> Sum/1
  Creating    qbar / ps/1(qbar / ps) -> r2d6/1
  Bus Selector1/2 -> Creating    qbar / ps/2(V)  "<TAS>"
  r2d1/1 -> Gain/1, Sum1/1  "alpha"
  LF_state/1 -> Sum2/2
  Sum2/1 -> Gain2/1, Sum1/2
  coeff1/1 -> Sum/3
  Demux1/1 -> r2d1/1
  Gain2/1 -> Sum/2
  Gain/1 -> Sum2/1
  Gain1/1 -> LF_state/1
  Sum1/1 -> Gain1/1
  state/1 -> Bus Selector1/1
  Sum/1 -> delta_lef (deg)/1
  Selector/1 -> Creating    qbar / ps/1(alt)

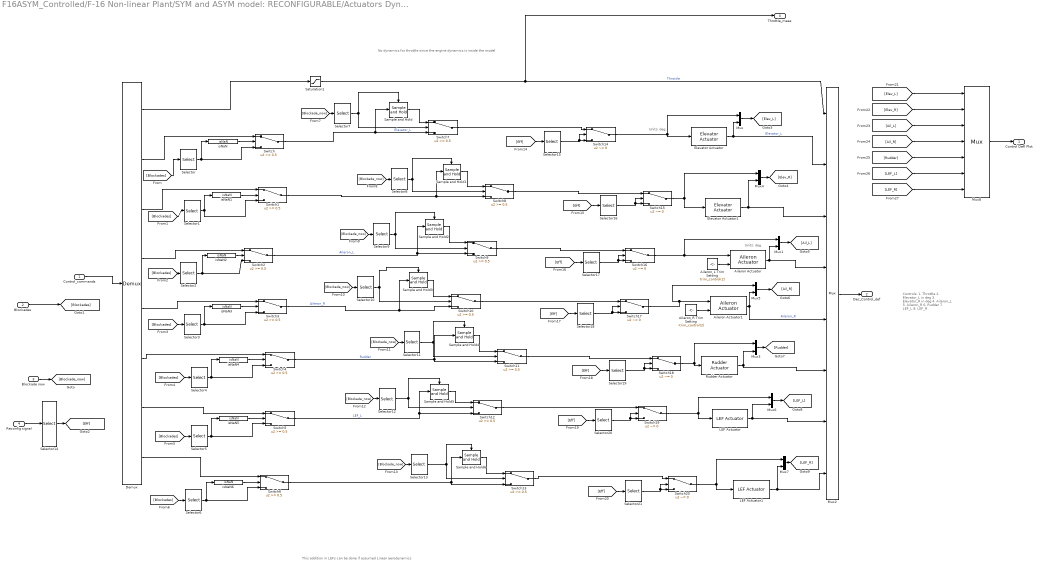
== system F16ASYM_Controlled/F-16 Non-linear Plant/SYM and ASYM model: RECONFIGURABLE/Actuators Dynamcis ==
  note: No dynamics for throttle since the engine dynamics is inside the model
  note: This addition in LEFs can be done
      |  if assumed Linear aerodynamics
  note: Units: deg.
  note: Units: deg.
  note: Controls:
      | 1. Throttle
      | 2. Elevator_L in deg
      | 3. Elevator_R in deg
      | 4. Aileron_L
      | 5. Aileron_R
      | 6. Rudder
      | 7. LEF_L
      | 8. LEF_R
  Control_commands : Inport
  Blockades : Inport  Port=2
  Blockade now : Inport  Port=3
  Reconfig signal : Inport  Port=4
  Aileron Actuator : F16_Actuator_Library/Aileron Actuator
  Aileron Actuator1 : F16_Actuator_Library/Aileron Actuator
  Aileron_L Trim Setting : Constant  Value=trim_control(2)
  Aileron_R Trim Setting : Constant  Value=-trim_control(2)
  Demux : Demux  Outputs=8
  Elevator Actuator : F16_Actuator_Library/Elevator Actuator
  Elevator Actuator1 : F16_Actuator_Library/Elevator Actuator
  LEF Actuator : F16_Actuator_Library/LEF Actuator
  LEF Actuator1 : F16_Actuator_Library/LEF Actuator
  Mux{,1,3..7} (7 alike) : Mux  Inputs=2
  Mux2 : Mux  Inputs=8
  Mux8 : Mux  Inputs=7
  Rudder Actuator : F16_Actuator_Library/Rudder Actuator
  Sample and Hold : dspsigops/Sample and Hold  trig=Rising edge  initCond=trim_control(1)  latchinput=off
  Sample and Hold1 : dspsigops/Sample and Hold  trig=Rising edge  initCond=trim_control(1)  latchinput=off
  Sample and Hold2 : dspsigops/Sample and Hold  trig=Rising edge  initCond=trim_control(2)  latchinput=off
  Sample and Hold3 : dspsigops/Sample and Hold  trig=Rising edge  initCond=-trim_control(2)  latchinput=off
  Sample and Hold4 : dspsigops/Sample and Hold  trig=Rising edge  initCond=trim_control(3)  latchinput=off
  Sample and Hold5 : dspsigops/Sample and Hold  trig=Rising edge  initCond=dLEF  latchinput=off
  Sample and Hold6 : dspsigops/Sample and Hold  trig=Rising edge  initCond=dLEF  latchinput=off
  Saturation1 : Saturate  UpperLimit=1  LowerLimit=0
  Selector : Selector  InputPortWidth=7
  Selector1 : Selector  InputPortWidth=7  Indices=2
  Selector10 : Selector  InputPortWidth=7  Indices=4
  Selector11 : Selector  InputPortWidth=7  Indices=5
  Selector12 : Selector  InputPortWidth=7  Indices=6
  Selector13 : Selector  InputPortWidth=7  Indices=7
  Selector14 : Selector  InputPortWidth=19  Indices=10:16
  Selector15 : Selector  InputPortWidth=7
  Selector16 : Selector  InputPortWidth=7  Indices=2
  Selector17 : Selector  InputPortWidth=7  Indices=3
  Selector18 : Selector  InputPortWidth=7  Indices=4
  Selector19 : Selector  InputPortWidth=7  Indices=5
  Selector2 : Selector  InputPortWidth=7  Indices=3
  Selector20 : Selector  InputPortWidth=7  Indices=6
  Selector21 : Selector  InputPortWidth=7  Indices=7
  Selector3 : Selector  InputPortWidth=7  Indices=4
  Selector4 : Selector  InputPortWidth=7  Indices=5
  Selector5 : Selector  InputPortWidth=7  Indices=6
  Selector6 : Selector  InputPortWidth=7  Indices=7
  Selector7 : Selector  InputPortWidth=7
  Selector8 : Selector  InputPortWidth=7  Indices=2
  Selector9 : Selector  InputPortWidth=7  Indices=3
  Switch{,1..13} (14 alike) : Switch  Threshold=0.5
  Switch{14..20} (7 alike) : Switch  Criteria=u2 ~= 0
  isNaN{,1..6} (7 alike) : RelationalOperator  Operator=isNaN  OutDataTypeStr=boolean
  Control Defl Plot : Outport
  Dec_Control_def : Outport  Port=2
  Throttle_meas : Outport  Port=3
  wires:
  Control_commands/1 -> Demux/1
  Switch14/1 -> Elevator Actuator/1, Mux/1
  Mux2/1 -> Dec_Control_def/1
  Switch16/1 -> Mux1/1, Aileron Actuator/1
  Switch18/1 -> Mux3/1, Rudder Actuator/1
  Switch19/1 -> Mux6/1, LEF Actuator/1
  Switch20/1 -> Mux7/1, LEF Actuator1/1
  Demux/1 -> Saturation1/1
  Aileron_L Trim Setting/1 -> Aileron Actuator/2
  Aileron_R Trim Setting/1 -> Aileron Actuator1/2
  Saturation1/1 -> Mux2/1, Throttle_meas/1  "Throttle"
  Blockades/1 -> [Blockades]
  Blockade now/1 -> [Blockade_now]
  [Blockades] -> Selector/1
  isNaN/1 -> Switch/2
  Demux/2 -> Switch/1
  Selector/1 -> Switch/3, isNaN/1
  [Blockades] -> Selector1/1
  isNaN1/1 -> Switch1/2
  Demux/3 -> Switch1/1
  Selector1/1 -> Switch1/3, isNaN1/1
  [Blockades] -> Selector2/1
  isNaN2/1 -> Switch2/2
  Demux/4 -> Switch2/1
  Selector2/1 -> Switch2/3, isNaN2/1
  [Blockades] -> Selector3/1
  isNaN3/1 -> Switch3/2
  Demux/5 -> Switch3/1
  Selector3/1 -> Switch3/3, isNaN3/1
  [Blockades] -> Selector4/1
  isNaN4/1 -> Switch4/2
  Demux/6 -> Switch4/1
  Selector4/1 -> Switch4/3, isNaN4/1
  [Blockades] -> Selector5/1
  isNaN5/1 -> Switch5/2
  Demux/7 -> Switch5/1
  Selector5/1 -> Switch5/3, isNaN5/1
  [Blockades] -> Selector6/1
  isNaN6/1 -> Switch6/2
  Demux/8 -> Switch6/1
  Selector6/1 -> Switch6/3, isNaN6/1
  Aileron Actuator/1 -> Mux2/4, Mux1/2
  Rudder Actuator/1 -> Mux3/2, Mux2/6
  LEF Actuator/1 -> Mux2/7, Mux6/2
  Switch/1 -> Switch7/3, Sample and Hold/1  "Elevator_L"
  [Blockade_now] -> Selector7/1
  Sample and Hold/1 -> Switch7/1
  Selector7/1 -> Switch7/2, Sample and Hold/Trigger
  Elevator Actuator/1 -> Mux/2, Mux2/2  "Elevator_L"
  Switch1/1 -> Sample and Hold1/1, Switch8/3
  [Blockade_now] -> Selector8/1
  Sample and Hold1/1 -> Switch8/1
  Selector8/1 -> Switch8/2, Sample and Hold1/Trigger
  Switch15/1 -> Mux4/1, Elevator Actuator1/1
  Switch2/1 -> Sample and Hold2/1, Switch9/3  "Aileron_L"
  [Blockade_now] -> Selector9/1
  Sample and Hold2/1 -> Switch9/1
  Selector9/1 -> Sample and Hold2/Trigger, Switch9/2
  Switch17/1 -> Mux5/1, Aileron Actuator1/1
  Aileron Actuator1/1 -> Mux2/5, Mux5/2  "Aileron_R"
  Switch3/1 -> Switch10/3, Sample and Hold3/1  "Aileron_R"
  [Blockade_now] -> Selector10/1
  Sample and Hold3/1 -> Switch10/1
  Selector10/1 -> Sample and Hold3/Trigger, Switch10/2
  Switch4/1 -> Switch11/3, Sample and Hold4/1  "Rudder"
  [Blockade_now] -> Selector11/1
  Sample and Hold4/1 -> Switch11/1
  Selector11/1 -> Switch11/2, Sample and Hold4/Trigger
  Switch5/1 -> Sample and Hold5/1, Switch12/3  "LEF_L"
  [Blockade_now] -> Selector12/1
  Sample and Hold5/1 -> Switch12/1
  Selector12/1 -> Switch12/2, Sample and Hold5/Trigger
  LEF Actuator1/1 -> Mux7/2, Mux2/8
  Switch6/1 -> Switch13/3, Sample and Hold6/1
  [Blockade_now] -> Selector13/1
  Sample and Hold6/1 -> Switch13/1
  Selector13/1 -> Switch13/2, Sample and Hold6/Trigger
  Elevator Actuator1/1 -> Mux4/2, Mux2/3
  Reconfig signal/1 -> Selector14/1
  Selector14/1 -> [Eff]
  [Eff] -> Selector15/1
  Switch7/1 -> Switch14/1
  Selector15/1 -> Switch14/2, Switch14/3
  [Eff] -> Selector16/1
  Switch8/1 -> Switch15/1
  Selector16/1 -> Switch15/2, Switch15/3
  [Eff] -> Selector17/1
  Switch9/1 -> Switch16/1
  Selector17/1 -> Switch16/2, Switch16/3
  [Eff] -> Selector18/1
  Switch10/1 -> Switch17/1
  Selector18/1 -> Switch17/2, Switch17/3
  [Eff] -> Selector19/1
  Switch11/1 -> Switch18/1
  Selector19/1 -> Switch18/2, Switch18/3
  [Eff] -> Selector20/1
  Switch12/1 -> Switch19/1
  Selector20/1 -> Switch19/2, Switch19/3
  [Eff] -> Selector21/1
  Switch13/1 -> Switch20/1
  Selector21/1 -> Switch20/2, Switch20/3
  Mux/1 -> [Elev_L]
  Mux4/1 -> [Elev_R]
  Mux1/1 -> [Ail_L]
  Mux5/1 -> [Ail_R]
  Mux3/1 -> [Rudder]
  Mux6/1 -> [LEF_L]
  Mux7/1 -> [LEF_R]
  Mux8/1 -> Control Defl Plot/1
  [Elev_L] -> Mux8/1
  [Elev_R] -> Mux8/2
  [Ail_L] -> Mux8/3
  [Ail_R] -> Mux8/4
  [Rudder] -> Mux8/5
  [LEF_L] -> Mux8/6
  [LEF_R] -> Mux8/7

== system F16ASYM_Controlled/F-16 Non-linear Plant/SYM and ASYM model: RECONFIGURABLE/Leading Edge Flap:Symetric deflection ==
  note: see NASA Technical Paper 1538, p34
  note: Same as atmos() in nlplant...c
  note: Initialize LF_state with -alpha0 value in degrees!!!!
  state : Inport
  Bus Selector1 : BusSelector  OutputSignals=X_e,TAS,alpha ; beta
  Creating    qbar / ps : Subsystem
  Gain : Gain  Gain=2  SaturateOnIntegerOverflow=on  OutDataTypeStr=Inherit: Same as input  ParamDataTypeStr=Inherit: Same as input
  Gain1 : Gain  Gain=7.25  SaturateOnIntegerOverflow=on  OutDataTypeStr=Inherit: Same as input  ParamDataTypeStr=Inherit: Same as input
  Gain2 : Gain  Gain=1.38  SaturateOnIntegerOverflow=on  OutDataTypeStr=Inherit: Same as input  ParamDataTypeStr=Inherit: Same as input
  LF_state : Integrator  InitialCondition=-trim_state(8)*180/pi
  Selector : Selector  InputPortWidth=3  Indices=3
  Selector1 : Selector  InputPortWidth=2
  Sum : Sum  Inputs=-|+|+  SaturateOnIntegerOverflow=on  InputSameDT=on  OutDataTypeStr=Inherit: Same as first input
  Sum1 : Sum  Inputs=|+-  SaturateOnIntegerOverflow=on  InputSameDT=on  OutDataTypeStr=Inherit: Same as first input
  Sum2 : Sum  Inputs=++|  SaturateOnIntegerOverflow=on  InputSameDT=on  OutDataTypeStr=Inherit: Same as first input
  coeff1 : Constant  Value=1.45
  r2d1 : Gain  Gain=180/pi  SaturateOnIntegerOverflow=on  OutDataTypeStr=Inherit: Same as input  ParamDataTypeStr=Inherit: Same as input
  r2d6 : Gain  Gain=9.05  SaturateOnIntegerOverflow=on  OutDataTypeStr=Inherit: Same as input  ParamDataTypeStr=Inherit: Same as input
  delta_lef (deg) : Outport
  wires:
  Sum/1 -> delta_lef (deg)/1
  state/1 -> Bus Selector1/1
  Sum1/1 -> Gain1/1
  Gain1/1 -> LF_state/1
  Gain/1 -> Sum2/1
  Gain2/1 -> Sum/2
  Selector1/1 -> r2d1/1
  coeff1/1 -> Sum/3
  Sum2/1 -> Sum1/2, Gain2/1
  LF_state/1 -> Sum2/2
  r2d1/1 -> Sum1/1, Gain/1  "alpha"
  Bus Selector1/2 -> Creating    qbar / ps/2(V)  "<TAS>"
  Creating    qbar / ps/1(qbar / ps) -> r2d6/1
  r2d6/1 -> Sum/1
  Bus Selector1/3 -> Selector1/1  "<alpha ; beta>"
  Bus Selector1/1 -> Selector/1  "<X_e>"
  Selector/1 -> Creating    qbar / ps/1(alt)

== system F16ASYM_Controlled/NDI/NDI: NO RECONFIG/Dim_less ==
  L_comm : Inport
  M_comm : Inport  Port=2
  N_comm : Inport  Port=3
  q : Inport  Port=4
  B span : Constant  Value=9.144
  CMA : Constant  Value=3.45
  Divide : Product  Inputs=*/
  Divide1 : Product  Inputs=***
  Divide2 : Product  Inputs=/*
  Divide3 : Product  Inputs=***
  Divide4 : Product  Inputs=*/
  S_w : Constant  Value=27.87
  S_w1 : Constant  Value=27.87
  q1 : InportShadow  Port=4
  C_L des : Outport
  C_M des : Outport  Port=2
  C_N des : Outport  Port=3
  wires:
  Divide4/1 -> C_M des/1  "C_M"
  Divide3/1 -> Divide4/2
  M_comm/1 -> Divide4/1
  CMA/1 -> Divide3/3
  S_w1/1 -> Divide3/2
  q1/1 -> Divide3/1
  Divide2/1 -> C_N des/1  "C_N"
  N_comm/1 -> Divide2/2
  Divide/1 -> C_L des/1  "C_L"
  Divide1/1 -> Divide/2, Divide2/1
  L_comm/1 -> Divide/1
  B span/1 -> Divide1/3
  S_w/1 -> Divide1/2
  q/1 -> Divide1/1

== system F16ASYM_Controlled/NDI/NDI: RECONFIG/Dim_less ==
  L_comm : Inport
  M_comm : Inport  Port=2
  N_comm : Inport  Port=3
  q : Inport  Port=4
  B span : Constant  Value=9.144
  CMA : Constant  Value=3.45
  Divide : Product  Inputs=*/
  Divide1 : Product  Inputs=***
  Divide2 : Product  Inputs=/*
  Divide3 : Product  Inputs=***
  Divide4 : Product  Inputs=*/
  S_w : Constant  Value=27.87
  S_w1 : Constant  Value=27.87
  q1 : InportShadow  Port=4
  C_L des : Outport
  C_M des : Outport  Port=2
  C_N des : Outport  Port=3
  wires:
  q/1 -> Divide1/1
  S_w/1 -> Divide1/2
  B span/1 -> Divide1/3
  L_comm/1 -> Divide/1
  Divide1/1 -> Divide2/1, Divide/2
  Divide/1 -> C_L des/1  "C_L"
  N_comm/1 -> Divide2/2
  Divide2/1 -> C_N des/1  "C_N"
  q1/1 -> Divide3/1
  S_w1/1 -> Divide3/2
  CMA/1 -> Divide3/3
  M_comm/1 -> Divide4/1
  Divide3/1 -> Divide4/2
  Divide4/1 -> C_M des/1  "C_M"
